simulink model "test_v1"  (R2019b)
settings: Solver=ode4  StartTime=0.0  StopTime=100  FixedStep=1e-3
libraries: simulink x2
settings Model: Creator=bitgar  LastModifiedBy=bitgar

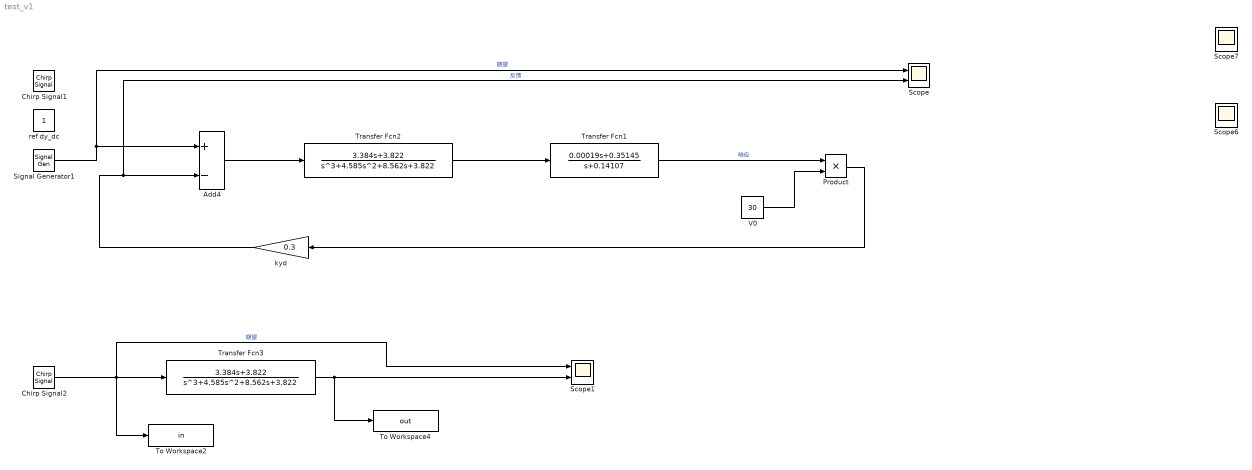
== system test_v1 ==
  Add4 : Sum  Inputs=+-
  Chirp Signal1 : simulink/Sources/Chirp Signal  f1=0.001  T=100  f2=2.5
  Chirp Signal2 : simulink/Sources/Chirp Signal  f1=0.001  T=100  f2=2.5
  Product : Product
  Scope{,1,6..7} (4 alike) : Scope  NumInputPorts=2
  Signal Generator1 : SignalGenerator  Frequency=0.0334
  To Workspace2 : ToWorkspace  VariableName=in  SampleTime=-1
  To Workspace4 : ToWorkspace  VariableName=out  SampleTime=-1
  Transfer Fcn1 : TransferFcn  Numerator=[0.00019 0.35145]  Denominator=[1 0.14107]
  Transfer Fcn2 : TransferFcn  Numerator=[3.384 3.822]  Denominator=[1 4.585 8.562 3.822]
  Transfer Fcn3 : TransferFcn  Numerator=[3.384 3.822]  Denominator=[1 4.585 8.562 3.822]
  V0 : Constant  Value=30
  kyd : Gain  Gain=0.3
  ref dy_dc : Constant
  wires:
  ? -> ?
  Transfer Fcn1/1 -> Product/1  "响应"
  Signal Generator1/1 -> Scope/1, Add4/1  "期望"
  kyd/1 -> Add4/2, Scope/2  "反馈"
  V0/1 -> Product/2
  Product/1 -> kyd/1
  Add4/1 -> Transfer Fcn2/1
  Transfer Fcn2/1 -> Transfer Fcn1/1
  Chirp Signal2/1 -> To Workspace2/1, Scope1/1, Transfer Fcn3/1  "期望"
  Transfer Fcn3/1 -> To Workspace4/1, Scope1/2
